simulink model "Trolley_Pendulum_RBF_Supervisory"  (R2023b)
settings: Solver=ode1  StartTime=0.0  StopTime=10  FixedStep=0.001  RelTol=1e-3
values from neighbouring files (symbols this model uses):
  E = C'*Q_bar*M    [inverted_pendulum.m]
  H = C'*Q_bar*C+R_bar    [inverted_pendulum.m]
  m_A_continue = double(subs(A_syms, [M, m, g, J, L, b], [M_, m_, g_, J_, L_, b_]))    [inverted_pendulum.m]
  m_B_continue = double(subs(B_syms, [M, m, g, J, L, b], [M_, m_, g_, J_, L_, b_]))    [inverted_pendulum.m]
  m_C_continue = C_syms    [inverted_pendulum.m]
  N = 20    [inverted_pendulum.m]
  Time_Step = 0.03    [inverted_pendulum.m]
  X = [x, x_dt, fai, fai_dt]    [inverted_pendulum.m]
  Y = [x, x_dt, fai, fai_dt]    [inverted_pendulum.m]
undefined symbols (not defined in the file or in its folder): K, Z
libraries: sm_lib x16, nesl_utility x6, rllib x1
settings Model: Creator=Lenovo  LastModifiedBy=15324
settings SolverCC: AlgebraicLoopSolver=TrustRegion
settings DataIOCC: LimitDataPoints=on  SaveFormat=Array  ReturnWorkspaceOutputs=off
settings OptimizationCC: BlockReduction=off  BooleanDataType=off  LifeSpan=inf
settings DebuggingCC: SaveWithParameterizedLinksMsg=none  UnderspecifiedInitializationDetection=Classic  MergeDetectMultiDrivingBlocksExec=none  SignalResolutionControl=TryResolveAllWithWarning  UnconnectedInputMsg=warning  UnconnectedOutputMsg=warning  UnconnectedLineMsg=warning  SFUnexpectedBacktrackingDiag=warning  SFNoUnconditionalDefaultTransitionDiag=warning  SFExecutionAtInitializationDiag=none  ArithmeticOperatorsInVariantConditions=warning
settings HardwareCC: ProdBitPerPointer=32  ProdBitPerSizeT=32  ProdBitPerPtrDiffT=32  ProdLargestAtomicFloat=None  ProdIntDivRoundTo=Undefined  ProdEndianess=Unspecified  ProdWordSize=32  ProdHWDeviceType=32-bit Generic  TargetUnknown=on
settings ModelReferenceCC: EnableRefExpFcnMdlSchedulingChecks=on  PropagateSignalLabelsOutOfModel=off
settings SFSimCC: SimUseLocalCustomCode=off  CustomCodeUndefinedFunction=UseInterfaceOnly
settings RTWCC: RTWUseLocalCustomCode=off
settings CodeAppCC: StateflowObjectComments=on
settings GRTTargetCC: TargetLangStandard=C89/C90 (ANSI)
settings ConfigComp: CovMetricSettings=dw  CovSaveCumulativeToWorkspaceVar=on  CovSaveSingleToWorkspaceVar=on  CovExternalEMLEnable=off

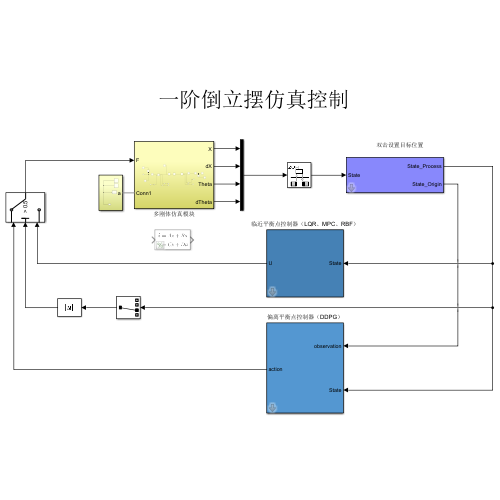
[thumbnail: Simulink's stored preview of the top-level diagram]
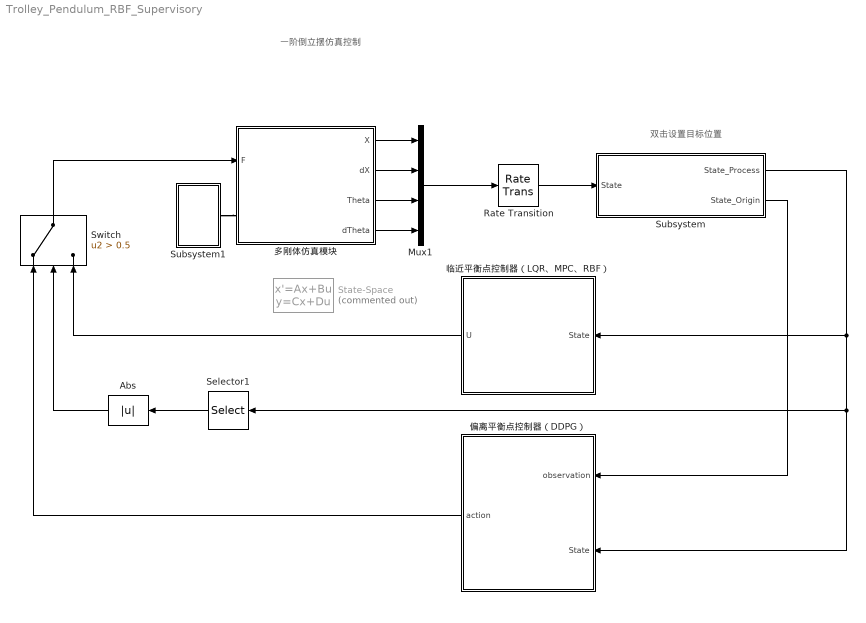
== system Trolley_Pendulum_RBF_Supervisory ==
  note: 双击设置目标位置
  note: 一阶倒立摆仿真控制
  Abs : Abs  SaturateOnIntegerOverflow=off
  Mux1 : Mux
  Rate Transition : RateTransition  OutPortSampleTime=Time_Step
  Selector1 : Selector  InputPortWidth=4  IndexOptions=Index vector (dialog)  Indices=[3]  OutputSizes=1
  State-Space : StateSpace  Commented=on  A=m_A_continue  B=m_B_continue  C=m_C_continue  D=[0;0;0;0]  InitialCondition=[0.5;0.5;0.5;0.5]
  Subsystem : Subsystem  mask{X_Target=1}
      mask prompts: X_Target "目标位置"
      mask DialogControl Set Prompt: 设置
  Subsystem1 : Subsystem
  Switch : Switch  Criteria=u2 > Threshold  Threshold=0.5  SaturateOnIntegerOverflow=off  InputSameDT=off
  临近平衡点控制器（LQR、MPC、RBF） : Subsystem  mask{MODE=MPC}
      mask prompts: MODE "模式设置"
      mask TypeOptions MODE: MPC | LQR | RBF
      mask DialogControl ParameterGroupVar Prompt: 设置
      mask DialogControl MODE Tooltip: A
  偏离平衡点控制器（DDPG） : Subsystem
      mask DialogControl ParameterGroupVar Prompt: 基于强化学习DDPG控制器
  多刚体仿真模块 : Subsystem
  wires:
  多刚体仿真模块/2(dX) -> Mux1/2
  Mux1/1 -> Rate Transition/1
  多刚体仿真模块/4(dTheta) -> Mux1/4
  多刚体仿真模块/1(X) -> Mux1/1
  多刚体仿真模块/3(Theta) -> Mux1/3
  Abs/1 -> Switch/2
  Selector1/1 -> Abs/1
  Switch/1 -> 多刚体仿真模块/1(F)
  Subsystem/1(State_Process) -> 偏离平衡点控制器（DDPG）/2(State), Selector1/1, 临近平衡点控制器（LQR、MPC、RBF）/1(State)
  Rate Transition/1 -> Subsystem/1(State)
  偏离平衡点控制器（DDPG）/1(action) -> Switch/1
  Subsystem/2(State_Origin) -> 偏离平衡点控制器（DDPG）/1(observation)
  临近平衡点控制器（LQR、MPC、RBF）/1(U) -> Switch/3
  connections:
  Subsystem1/RConn1 -- 多刚体仿真模块/LConn1

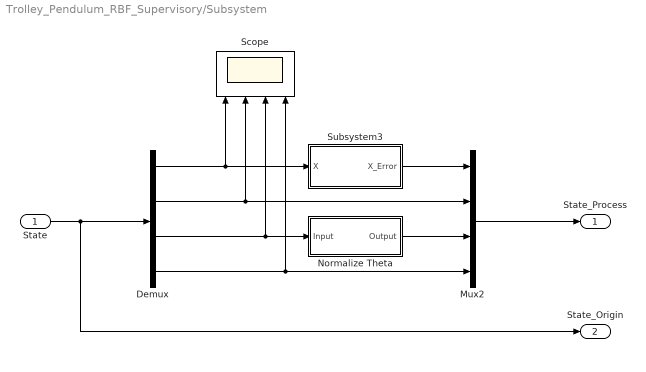
== system Trolley_Pendulum_RBF_Supervisory/Subsystem ==
  State : Inport
  Demux : Demux
  Mux2 : Mux
  Normalize Theta : Subsystem
  Scope : Scope  NumInputPorts=4
  Subsystem3 : Subsystem  mask{POS_REF=X_Target}
      mask prompts: POS_REF "目标位置"
      mask DialogControl ParameterGroupVar Prompt: 参数
  State_Process : Outport
  State_Origin : Outport  Port=2
  wires:
  Mux2/1 -> State_Process/1
  State/1 -> State_Origin/1, Demux/1
  Demux/2 -> Scope/2, Mux2/2
  Normalize Theta/1(Output) -> Mux2/3
  Demux/3 -> Scope/3, Normalize Theta/1(Input)
  Demux/4 -> Scope/4, Mux2/4
  Demux/1 -> Scope/1, Subsystem3/1(X)
  Subsystem3/1(X_Error) -> Mux2/1

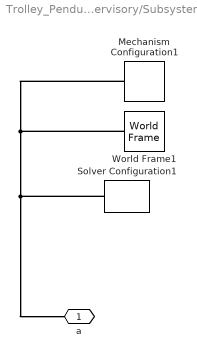
== system Trolley_Pendulum_RBF_Supervisory/Subsystem1 ==
  Mechanism Configuration1 : sm_lib/Utilities/Mechanism Configuration  UniformGravity=Constant  GravityVector=[0 0 -9.80665]  GravityVectorUnits=m/s^2  LinearizationDelta=0.0001  JointModeTransitionNonlinearIterations=2
  Solver Configuration1 : nesl_utility/Solver Configuration  PhysicalDomain=network_engine_domain  SubClassName=solver  LeftPortType=input  RightPortType=generic  Tones=[]  Harmonics=[]  SimulateNoise=off  Profile=off  UseLocalSampling=off  EnableSwitchedLinearOptims=on  FrequencyDomain=off  UseCCode=off  RelTol=0.001  AbsTol=1e-06  MinStep=1e-09  ToWorkspace=off  RevertToSquareIcSolve=off  NumHomotopyIterations=100  PhasorMode=off  PhasorModeNumHarmonics=1  ConsistencySolver=NEWTON_FTOL  IndexReductionMethod=DerivativeReplacement  DoDC=off  ResidualTolerance=1e-09  ConsistencyTolSource=GLOBAL  ConsistencyAbsTol=0.001  ConsistencyRelTol=0.001  ConsistencyTolFactor=0.001  UseLocalSolver=off  LocalSolverChoice=NE_BACKWARD_EULER_ADVANCER  ResolveIndetEquations=on  FunctionEvalNumThread=1  LocalSolverSampleTime=0.001  DoFixedCost=off  MaxNonlinIter=3  MaxModeIter=2  ComputeImpulses=off  ImpulseIterations=2  LinearAlgebra=auto  LinearAlgebraNumThread=0  EquationFormulation=NE_TIME_EF  DelaysMemoryBudget=1024  AutomaticFiltering=on  FilteringTimeConstant=0.001  PartitionStorageMethod=AS_NEEDED  PartitionMemoryBudget=1024  PartitionMethod=ROBUST  MultibodyUseLocalSolver=off  MultibodyLocalSolverChoice=ODE1  MultibodyLocalSolverSampleTime=0.001
  World Frame1 : sm_lib/Frames and Transforms/World Frame
  a : PMIOPort  Side=Right
  connections:
  Mechanism Configuration1/RConn1 -- a/RConn1 -- Solver Configuration1/RConn1 -- World Frame1/RConn1

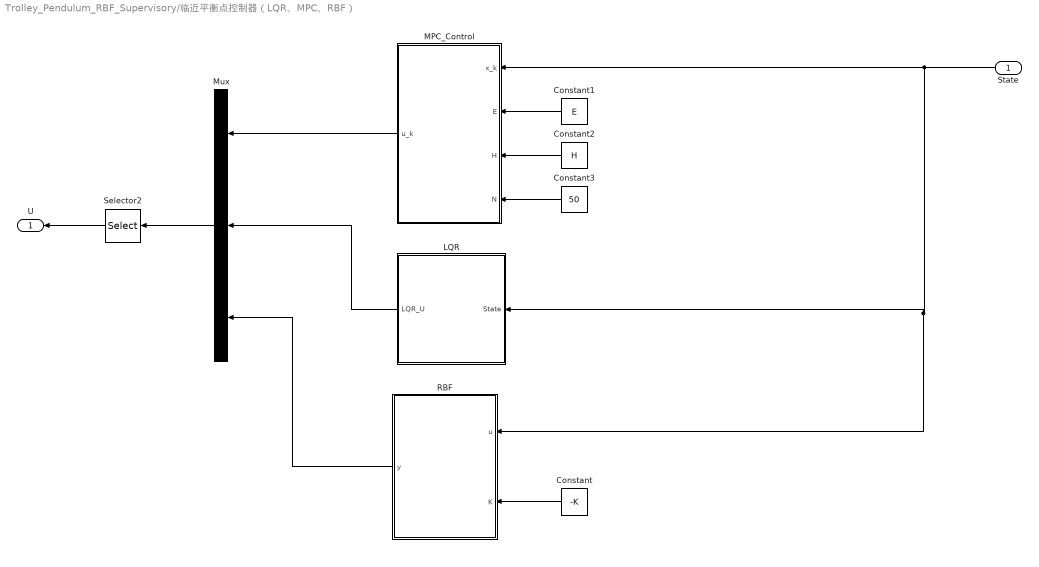
== system Trolley_Pendulum_RBF_Supervisory/临近平衡点控制器（LQR、MPC、RBF） ==
  State : Inport
  Constant : Constant  Value=-K  VectorParams1D=off
  Constant1 : Constant  Value=E  VectorParams1D=off
  Constant2 : Constant  Value=H  VectorParams1D=off
  Constant3 : Constant  Value=50
  LQR : Subsystem  mask{LQR_K=K}
      mask prompts: LQR_K "LQR_K矩阵"
      mask DialogControl ParameterGroupVar Prompt: 参数
  MPC_Control : MATLAB Function  TreatAsAtomicUnit=on
  Mux : Mux  Inputs=3
  RBF : MATLAB Function  TreatAsAtomicUnit=on
  Selector2 : Selector  InputPortWidth=3  IndexOptions=Index vector (dialog)  Indices=[MODE]  OutputSizes=1
  U : Outport
  wires:
  Selector2/1 -> U/1
  LQR/1(LQR_U) -> Mux/2
  MPC_Control/1(u_k) -> Mux/1
  Mux/1 -> Selector2/1
  Constant1/1 -> MPC_Control/2(E)
  Constant/1 -> RBF/2(K)
  RBF/1(y) -> Mux/3
  Constant2/1 -> MPC_Control/3(H)
  Constant3/1 -> MPC_Control/4(N)
  State/1 -> RBF/1(u), LQR/1(State), MPC_Control/1(x_k)

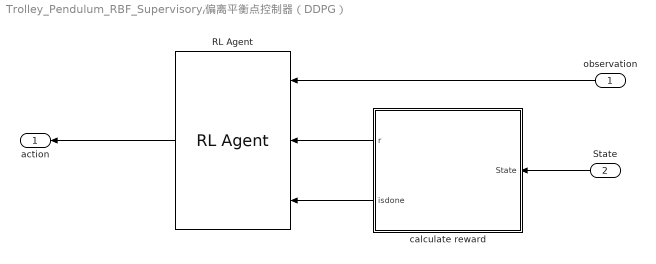
== system Trolley_Pendulum_RBF_Supervisory/偏离平衡点控制器（DDPG） ==
  observation : Inport
  State : Inport  Port=2
  RL Agent : rllib/RL Agent  Agent=saved_agent  ExternalActionAsInput=off  ProvideLastAction=off  ProvideCumRwd=off  TreatAsDirectFeedthrough=on  UseStrictObservationDataTypes=off
  calculate reward : Subsystem
  action : Outport
  wires:
  observation/1 -> RL Agent/1
  calculate reward/2(isdone) -> RL Agent/3
  calculate reward/1(r) -> RL Agent/2
  State/1 -> calculate reward/1(State)
  RL Agent/1 -> action/1

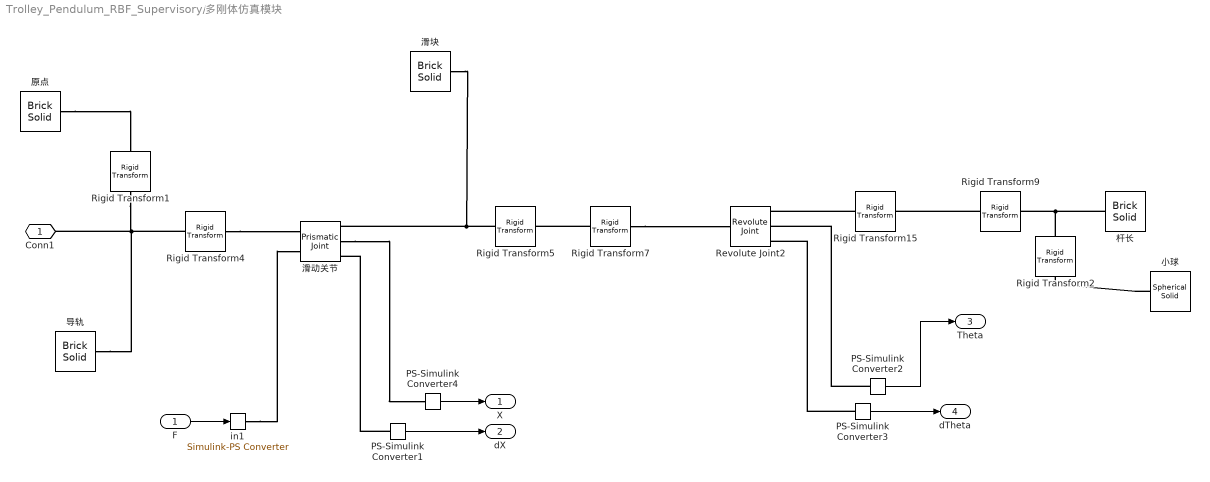
== system Trolley_Pendulum_RBF_Supervisory/多刚体仿真模块 ==
  F : Inport
  PS-Simulink Converter1 : nesl_utility/PS-Simulink Converter  PhysicalDomain=network_engine_domain  SubClassName=ps_output  LeftPortType=input  RightPortType=output  PseudoPeriodic=off  Frequencies=[]  VectorFormat=inherit  Unit=m/s  AffineConversion=off
  PS-Simulink Converter2 : nesl_utility/PS-Simulink Converter  PhysicalDomain=network_engine_domain  SubClassName=ps_output  LeftPortType=input  RightPortType=output  PseudoPeriodic=off  Frequencies=[]  VectorFormat=inherit  Unit=rad  AffineConversion=off
  PS-Simulink Converter3 : nesl_utility/PS-Simulink Converter  PhysicalDomain=network_engine_domain  SubClassName=ps_output  LeftPortType=input  RightPortType=output  PseudoPeriodic=off  Frequencies=[]  VectorFormat=inherit  Unit=rad/s  AffineConversion=off
  PS-Simulink Converter4 : nesl_utility/PS-Simulink Converter  PhysicalDomain=network_engine_domain  SubClassName=ps_output  LeftPortType=input  RightPortType=output  PseudoPeriodic=off  Frequencies=[]  VectorFormat=inherit  Unit=m  AffineConversion=off
  Revolute Joint2 : sm_lib/Joints/Revolute Joint  JointMode=Normal  SenseConstraintForce=off  SenseConstraintForceX=off  SenseConstraintForceY=off  SenseConstraintForceZ=off  SenseConstraintTorque=off  SenseConstraintTorqueX=off  SenseConstraintTorqueY=off  SenseConstraintTorqueZ=off  SenseTotalForce=off  SenseTotalForceX=off  SenseTotalForceY=off  SenseTotalForceZ=off  SenseTotalTorque=off  SenseTotalTorqueX=off  SenseTotalTorqueY=off  SenseTotalTorqueZ=off  CompositeWrenchDir=FollowerOnBase  CompositeWrenchFrame=BaseFrame  EquilibriumPosition=0  EquilibriumPositionUnits=deg  SpringStiffness=0  SpringStiffnessUnits=N*m/deg  DampingCoefficient=0  DampingCoefficientUnits=N*m/(deg/s)  TorqueActuationMode=NoTorque  MotionActuationMode=ComputedMotion  SensePosition=on  SenseVelocity=on  SenseAcceleration=off  SenseTorqueForce=off  SenseLowerLimitTorqueForce=off  SenseUpperLimitTorqueForce=off  LowerLimitSpecify=off  LowerLimitBound=-90  LowerLimitBoundUnits=deg  LowerLimitStiffness=1e4  LowerLimitStiffnessUnits=N*m/deg  LowerLimitDamping=10  LowerLimitDampingUnits=N*m/(deg/s)  LowerLimitTransitionRegionWidth=0.1  LowerLimitTransitionRegionWidthUnits=deg  UpperLimitSpecify=off  UpperLimitBound=90  UpperLimitBoundUnits=deg  UpperLimitStiffness=1e4  UpperLimitStiffnessUnits=N*m/deg  UpperLimitDamping=10  UpperLimitDampingUnits=N*m/(deg/s)  UpperLimitTransitionRegionWidth=0.1  UpperLimitTransitionRegionWidthUnits=deg  PositionTargetSpecify=on  PositionTargetPriority=High  PositionTargetValue=150  PositionTargetValueUnits=deg  VelocityTargetSpecify=off  VelocityTargetPriority=High  VelocityTargetValue=0  VelocityTargetValueUnits=deg/s
  Rigid Transform1 : sm_lib/Frames and Transforms/Rigid Transform  TranslationMethod=None  TranslationStandardOffset=0  TranslationStandardOffsetUnits=m  TranslationStandardAxis=+Z  TranslationCartesianOffset=[0 0 0]  TranslationCartesianOffsetUnits=m  TranslationROffset=0  TranslationROffsetUnits=m  TranslationZOffset=0  TranslationZOffsetUnits=m  TranslationThetaOffset=0  TranslationThetaOffsetUnits=deg  RotationMethod=StandardAxis  RotationAngleUnits=deg  RotationStandardAxis=+Y  RotationAngle=90  RotationArbitraryAxis=[0 0 1]  FollAlignAxisA=+X  BaseAlignAxisA=+Y  FollAlignAxisB=+Y  BaseAlignAxisB=+Z  RotationSequenceAxes=FollowerAxes  RotationSequence=XYX  RotationSequenceAngles=[0 0 0]  RotationSequenceAnglesUnits=deg  RotationMatrix=[1 0 0; 0 1 0; 0 0 1]  Quaternion=[1 0 0 0]
  Rigid Transform15 : sm_lib/Frames and Transforms/Rigid Transform  TranslationMethod=None  TranslationStandardOffset=0  TranslationStandardOffsetUnits=m  TranslationStandardAxis=+Z  TranslationCartesianOffset=[0 0 0]  TranslationCartesianOffsetUnits=m  TranslationROffset=0  TranslationROffsetUnits=m  TranslationZOffset=0  TranslationZOffsetUnits=m  TranslationThetaOffset=0  TranslationThetaOffsetUnits=deg  RotationMethod=StandardAxis  RotationAngleUnits=deg  RotationStandardAxis=+X  RotationAngle=-90  RotationArbitraryAxis=[0 0 1]  FollAlignAxisA=+X  BaseAlignAxisA=+Y  FollAlignAxisB=+Y  BaseAlignAxisB=+Z  RotationSequenceAxes=FollowerAxes  RotationSequence=XYX  RotationSequenceAngles=[0 0 0]  RotationSequenceAnglesUnits=deg  RotationMatrix=[1 0 0; 0 1 0; 0 0 1]  Quaternion=[1 0 0 0]
  Rigid Transform2 : sm_lib/Frames and Transforms/Rigid Transform  TranslationMethod=StandardAxis  TranslationStandardOffset=25  TranslationStandardOffsetUnits=cm  TranslationStandardAxis=+Z  TranslationCartesianOffset=[0 0 0]  TranslationCartesianOffsetUnits=cm  TranslationROffset=0  TranslationROffsetUnits=m  TranslationZOffset=0  TranslationZOffsetUnits=m  TranslationThetaOffset=0  TranslationThetaOffsetUnits=deg  RotationMethod=None  RotationAngleUnits=deg  RotationStandardAxis=+X  RotationAngle=90  RotationArbitraryAxis=[0 0 1]  FollAlignAxisA=+X  BaseAlignAxisA=+Y  FollAlignAxisB=+Y  BaseAlignAxisB=+Z  RotationSequenceAxes=FollowerAxes  RotationSequence=XYX  RotationSequenceAngles=[0 0 0]  RotationSequenceAnglesUnits=deg  RotationMatrix=[1 0 0; 0 1 0; 0 0 1]  Quaternion=[1 0 0 0]
  Rigid Transform4 : sm_lib/Frames and Transforms/Rigid Transform  TranslationMethod=None  TranslationStandardOffset=0  TranslationStandardOffsetUnits=m  TranslationStandardAxis=+Z  TranslationCartesianOffset=[0 0 0]  TranslationCartesianOffsetUnits=m  TranslationROffset=0  TranslationROffsetUnits=m  TranslationZOffset=0  TranslationZOffsetUnits=m  TranslationThetaOffset=0  TranslationThetaOffsetUnits=deg  RotationMethod=StandardAxis  RotationAngleUnits=deg  RotationStandardAxis=+Y  RotationAngle=90  RotationArbitraryAxis=[0 0 1]  FollAlignAxisA=+X  BaseAlignAxisA=+Y  FollAlignAxisB=+Y  BaseAlignAxisB=+Z  RotationSequenceAxes=FollowerAxes  RotationSequence=XYX  RotationSequenceAngles=[0 0 0]  RotationSequenceAnglesUnits=deg  RotationMatrix=[1 0 0; 0 1 0; 0 0 1]  Quaternion=[1 0 0 0]
  Rigid Transform5 : sm_lib/Frames and Transforms/Rigid Transform  TranslationMethod=None  TranslationStandardOffset=0  TranslationStandardOffsetUnits=m  TranslationStandardAxis=+Z  TranslationCartesianOffset=[0 0 0]  TranslationCartesianOffsetUnits=m  TranslationROffset=0  TranslationROffsetUnits=m  TranslationZOffset=0  TranslationZOffsetUnits=m  TranslationThetaOffset=0  TranslationThetaOffsetUnits=deg  RotationMethod=StandardAxis  RotationAngleUnits=deg  RotationStandardAxis=+Y  RotationAngle=-90  RotationArbitraryAxis=[0 0 1]  FollAlignAxisA=+X  BaseAlignAxisA=+Y  FollAlignAxisB=+Y  BaseAlignAxisB=+Z  RotationSequenceAxes=FollowerAxes  RotationSequence=XYX  RotationSequenceAngles=[0 0 0]  RotationSequenceAnglesUnits=deg  RotationMatrix=[1 0 0; 0 1 0; 0 0 1]  Quaternion=[1 0 0 0]
  Rigid Transform7 : sm_lib/Frames and Transforms/Rigid Transform  TranslationMethod=None  TranslationStandardOffset=0  TranslationStandardOffsetUnits=m  TranslationStandardAxis=+Z  TranslationCartesianOffset=[0 0 0]  TranslationCartesianOffsetUnits=m  TranslationROffset=0  TranslationROffsetUnits=m  TranslationZOffset=0  TranslationZOffsetUnits=m  TranslationThetaOffset=0  TranslationThetaOffsetUnits=deg  RotationMethod=StandardAxis  RotationAngleUnits=deg  RotationStandardAxis=+X  RotationAngle=+90  RotationArbitraryAxis=[0 0 1]  FollAlignAxisA=+X  BaseAlignAxisA=+Y  FollAlignAxisB=+Y  BaseAlignAxisB=+Z  RotationSequenceAxes=FollowerAxes  RotationSequence=XYX  RotationSequenceAngles=[0 0 0]  RotationSequenceAnglesUnits=deg  RotationMatrix=[1 0 0; 0 1 0; 0 0 1]  Quaternion=[1 0 0 0]
  Rigid Transform9 : sm_lib/Frames and Transforms/Rigid Transform  TranslationMethod=StandardAxis  TranslationStandardOffset=25  TranslationStandardOffsetUnits=cm  TranslationStandardAxis=+Z  TranslationCartesianOffset=[0 0 0]  TranslationCartesianOffsetUnits=cm  TranslationROffset=0  TranslationROffsetUnits=m  TranslationZOffset=0  TranslationZOffsetUnits=m  TranslationThetaOffset=0  TranslationThetaOffsetUnits=deg  RotationMethod=None  RotationAngleUnits=deg  RotationStandardAxis=+X  RotationAngle=90  RotationArbitraryAxis=[0 0 1]  FollAlignAxisA=+X  BaseAlignAxisA=+Y  FollAlignAxisB=+Y  BaseAlignAxisB=+Z  RotationSequenceAxes=FollowerAxes  RotationSequence=XYX  RotationSequenceAngles=[0 0 0]  RotationSequenceAnglesUnits=deg  RotationMatrix=[1 0 0; 0 1 0; 0 0 1]  Quaternion=[1 0 0 0]
  in1 : nesl_utility/Simulink-PS Converter  PhysicalDomain=network_engine_domain  SubClassName=ps_input  LeftPortType=input  RightPortType=output  PseudoPeriodic=off  Frequencies=[]  NoiseDistribution=none  NoiseParameters=[]  Unit=1  AffineConversion=off  FilteringAndDerivatives=provide  SimscapeFilterOrder=1  InputFilterTimeConstant=0.001  UdotUserProvided=0
  原点 : sm_lib/Body Elements/Brick Solid  GraphicAmbientColor=[0.15 0.15 0.15 1.0]  BasedOnType=Density  BrickDimensions=[5 11 5]  BrickDimensionsUnits=cm  CenterOfMass=[0 0 0]  CenterOfMassUnits=m  GraphicDiffuseColor=[0.3 0.8 0.5]  Density=0.1  DensityUnits=g/cm^3  DoExposeReferenceFrame=on  GraphicEmissiveColor=[0.0 0.0 0.0 1.0]  ExportEntireGeometry=off  SerializedFrames=<Frames/>  MarkerShape=Sphere  MarkerSize=10  GraphicType=FromGeometry  InertiaType=CalculateFromGeometry  Mass=1  MassUnits=kg  MomentsOfInertia=[1 1 1]  MomentsOfInertiaUnits=kg*m^2  GraphicOpacity=1.0  ProductsOfInertia=[0 0 0]  ProductsOfInertiaUnits=kg*m^2  GraphicShininess=75  GraphicSpecularColor=[0.5 0.5 0.5 1.0]  GraphicVisPropType=SimpleVisualProperties
  导轨 : sm_lib/Body Elements/Brick Solid  GraphicAmbientColor=[0.15 0.15 0.15 1.0]  BasedOnType=Density  BrickDimensions=[500 5 5]  BrickDimensionsUnits=cm  CenterOfMass=[0 0 0]  CenterOfMassUnits=m  GraphicDiffuseColor=[0 0 0]  Density=0.1  DensityUnits=g/cm^3  DoExposeReferenceFrame=on  GraphicEmissiveColor=[0.0 0.0 0.0 1.0]  ExportEntireGeometry=off  SerializedFrames=<Frames/>  MarkerShape=Sphere  MarkerSize=10  GraphicType=FromGeometry  InertiaType=CalculateFromGeometry  Mass=1  MassUnits=kg  MomentsOfInertia=[1 1 1]  MomentsOfInertiaUnits=kg*m^2  GraphicOpacity=1.0  ProductsOfInertia=[0 0 0]  ProductsOfInertiaUnits=kg*m^2  GraphicShininess=75  GraphicSpecularColor=[0.5 0.5 0.5 1.0]  GraphicVisPropType=SimpleVisualProperties
  小球 : sm_lib/Body Elements/Spherical Solid  GraphicAmbientColor=[0.15 0.15 0.15 1.0]  BasedOnType=Density  CenterOfMass=[0 0 0]  CenterOfMassUnits=m  GraphicDiffuseColor=[0.5 0.8 0.5]  Density=1  DensityUnits=kg/m^3  DoExposeReferenceFrame=on  GraphicEmissiveColor=[0.0 0.0 0.0 1.0]  ExportEntireGeometry=off  SerializedExposedGeometries=<exposedGeometries/>  SerializedFrames=<Frames/>  MarkerShape=Sphere  MarkerSize=10  GraphicType=FromGeometry  InertiaType=CalculateFromGeometry  Mass=1  MassUnits=kg  MomentsOfInertia=[1 1 1]  MomentsOfInertiaUnits=kg*m^2  GraphicOpacity=1.0  ProductsOfInertia=[0 0 0]  ProductsOfInertiaUnits=kg*m^2  GraphicShininess=75  GraphicSpecularColor=[0.5 0.5 0.5 1.0]  SphereRadius=3.5  SphereRadiusUnits=cm  GraphicVisPropType=SimpleVisualProperties
  杆长 : sm_lib/Body Elements/Brick Solid  GraphicAmbientColor=[0.15 0.15 0.15 1.0]  BasedOnType=Density  BrickDimensions="[5 5  50]"  BrickDimensionsUnits=cm  CenterOfMass=[0 0 0]  CenterOfMassUnits=m  GraphicDiffuseColor=[0.8 0.5 0.1]  Density=1  DensityUnits=g/cm^3  DoExposeReferenceFrame=on  GraphicEmissiveColor=[0.0 0.0 0.0 1.0]  ExportEntireGeometry=off  SerializedFrames=<Frames/>  MarkerShape=Sphere  MarkerSize=10  GraphicType=FromGeometry  InertiaType=CalculateFromGeometry  Mass=1  MassUnits=kg  MomentsOfInertia=[1 1 1]  MomentsOfInertiaUnits=kg*m^2  GraphicOpacity=1.0  ProductsOfInertia=[0 0 0]  ProductsOfInertiaUnits=kg*m^2  GraphicShininess=75  GraphicSpecularColor=[0.5 0.5 0.5 1.0]  GraphicVisPropType=SimpleVisualProperties
  滑动关节 : sm_lib/Joints/Prismatic Joint  JointMode=Normal  SenseConstraintForce=off  SenseConstraintForceX=off  SenseConstraintForceY=off  SenseConstraintForceZ=off  SenseConstraintTorque=off  SenseConstraintTorqueX=off  SenseConstraintTorqueY=off  SenseConstraintTorqueZ=off  SenseTotalForce=off  SenseTotalForceX=off  SenseTotalForceY=off  SenseTotalForceZ=off  SenseTotalTorque=off  SenseTotalTorqueX=off  SenseTotalTorqueY=off  SenseTotalTorqueZ=off  CompositeWrenchDir=FollowerOnBase  CompositeWrenchFrame=BaseFrame  EquilibriumPosition=0  EquilibriumPositionUnits=m  SpringStiffness=0  SpringStiffnessUnits=N/m  DampingCoefficient=0  DampingCoefficientUnits=N/(m/s)  TorqueActuationMode=InputTorque  MotionActuationMode=ComputedMotion  SensePosition=on  SenseVelocity=on  SenseAcceleration=off  SenseTorqueForce=off  SenseLowerLimitTorqueForce=off  SenseUpperLimitTorqueForce=off  LowerLimitSpecify=off  LowerLimitBound=-1  LowerLimitBoundUnits=m  LowerLimitStiffness=1e6  LowerLimitStiffnessUnits=N/m  LowerLimitDamping=1e3  LowerLimitDampingUnits=N/(m/s)  LowerLimitTransitionRegionWidth=1e-4  LowerLimitTransitionRegionWidthUnits=m  UpperLimitSpecify=off  UpperLimitBound=1  UpperLimitBoundUnits=m  UpperLimitStiffness=1e6  UpperLimitStiffnessUnits=N/m  UpperLimitDamping=1e3  UpperLimitDampingUnits=N/(m/s)  UpperLimitTransitionRegionWidth=1e-4  UpperLimitTransitionRegionWidthUnits=m  PositionTargetSpecify=off  PositionTargetPriority=High  PositionTargetValue=0  PositionTargetValueUnits=m  VelocityTargetSpecify=off  VelocityTargetPriority=High  VelocityTargetValue=0  VelocityTargetValueUnits=m/s
  滑块 : sm_lib/Body Elements/Brick Solid  GraphicAmbientColor=[0.15 0.15 0.15 1.0]  BasedOnType=Density  BrickDimensions=[10 10 10]  BrickDimensionsUnits=cm  CenterOfMass=[0 0 0]  CenterOfMassUnits=m  GraphicDiffuseColor=[0.1 0.1 0.8]  Density=1  DensityUnits=g/cm^3  DoExposeReferenceFrame=on  GraphicEmissiveColor=[0.0 0.0 0.0 1.0]  ExportEntireGeometry=off  SerializedFrames=<Frames/>  MarkerShape=Sphere  MarkerSize=10  GraphicType=FromGeometry  InertiaType=CalculateFromGeometry  Mass=1  MassUnits=kg  MomentsOfInertia=[1 1 1]  MomentsOfInertiaUnits=kg*m^2  GraphicOpacity=1.0  ProductsOfInertia=[0 0 0]  ProductsOfInertiaUnits=kg*m^2  GraphicShininess=75  GraphicSpecularColor=[0.5 0.5 0.5 1.0]  GraphicVisPropType=SimpleVisualProperties
  Conn1 : PMIOPort  Side=Left
  X : Outport
  dX : Outport  Port=2
  Theta : Outport  Port=3
  dTheta : Outport  Port=4
  wires:
  F/1 -> in1/1
  PS-Simulink Converter1/1 -> dX/1
  PS-Simulink Converter3/1 -> dTheta/1
  PS-Simulink Converter2/1 -> Theta/1
  PS-Simulink Converter4/1 -> X/1
  connections:
  Rigid Transform9/LConn1 -- Rigid Transform15/RConn1
  in1/RConn1 -- 滑动关节/LConn2
  Rigid Transform15/LConn1 -- Revolute Joint2/RConn1
  Rigid Transform7/RConn1 -- Revolute Joint2/LConn1
  杆长/RConn1 -- Rigid Transform2/LConn1 -- Rigid Transform9/RConn1
  PS-Simulink Converter3/LConn1 -- Revolute Joint2/RConn3
  Rigid Transform7/LConn1 -- Rigid Transform5/RConn1
  Rigid Transform4/RConn1 -- 滑动关节/LConn1
  PS-Simulink Converter2/LConn1 -- Revolute Joint2/RConn2
  Rigid Transform4/LConn1 -- Rigid Transform1/RConn1 -- Conn1/RConn1 -- 导轨/RConn1
  PS-Simulink Converter1/LConn1 -- 滑动关节/RConn3
  滑动关节/RConn2 -- PS-Simulink Converter4/LConn1
  原点/RConn1 -- Rigid Transform1/LConn1
  小球/RConn1 -- Rigid Transform2/RConn1
  Rigid Transform5/LConn1 -- 滑块/RConn1 -- 滑动关节/RConn1

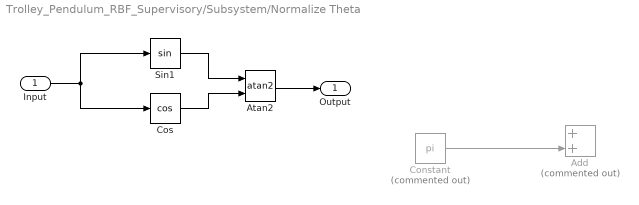
== system Trolley_Pendulum_RBF_Supervisory/Subsystem/Normalize Theta ==
  Input : Inport
  Add : Sum  Commented=on
  Atan2 : Trigonometry  Operator=atan2
  Constant : Constant  Commented=on  Value=pi
  Cos : Trigonometry  Operator=cos
  Sin1 : Trigonometry
  Output : Outport
  wires:
  Input/1 -> Cos/1, Sin1/1
  Sin1/1 -> Atan2/1
  Cos/1 -> Atan2/2
  Atan2/1 -> Output/1
  Constant/1 -> Add/2

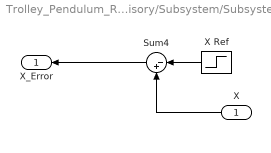
== system Trolley_Pendulum_RBF_Supervisory/Subsystem/Subsystem3 ==
  X : Inport
  Sum4 : Sum  Inputs=|-+
  X Ref : Step  Time=0  After=POS_REF  SampleTime=Time_Step
  X_Error : Outport
  wires:
  X Ref/1 -> Sum4/1
  X/1 -> Sum4/2
  Sum4/1 -> X_Error/1

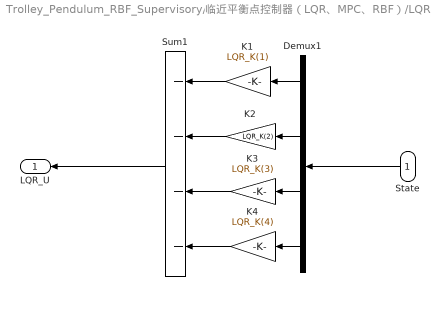
== system Trolley_Pendulum_RBF_Supervisory/临近平衡点控制器（LQR、MPC、RBF）/LQR ==
  State : Inport
  Demux1 : Demux
  K1 : Gain  Gain=LQR_K(1)
  K2 : Gain  Gain=LQR_K(2)
  K3 : Gain  Gain=LQR_K(3)
  K4 : Gain  Gain=LQR_K(4)
  Sum1 : Sum  Inputs=----
  LQR_U : Outport
  wires:
  K2/1 -> Sum1/2
  K1/1 -> Sum1/1
  K3/1 -> Sum1/3
  K4/1 -> Sum1/4
  Sum1/1 -> LQR_U/1
  State/1 -> Demux1/1
  Demux1/2 -> K2/1
  Demux1/3 -> K3/1
  Demux1/4 -> K4/1
  Demux1/1 -> K1/1

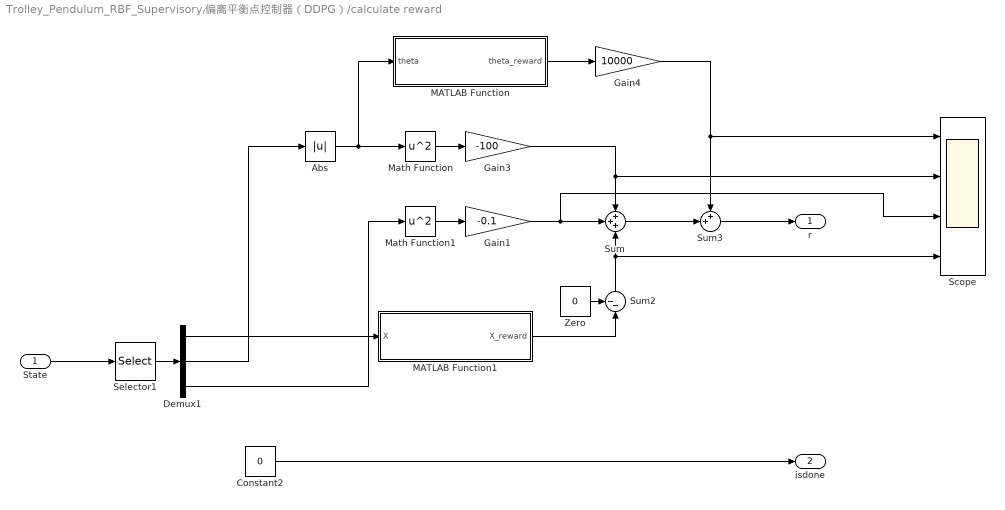
== system Trolley_Pendulum_RBF_Supervisory/偏离平衡点控制器（DDPG）/calculate reward ==
  State : Inport
  Abs : Abs  SaturateOnIntegerOverflow=off
  Constant2 : Constant  Value=0
  Demux1 : Demux  Outputs=3
  Gain1 : Gain  Gain=-0.1
  Gain3 : Gain  Gain=-100
  Gain4 : Gain  Gain=10000
  MATLAB Function : MATLAB Function  TreatAsAtomicUnit=on
  MATLAB Function1 : MATLAB Function  TreatAsAtomicUnit=on
  Math Function : Math  Operator=square  SignedPower=on
  Math Function1 : Math  Operator=square  SignedPower=on
  Scope : Scope  NumInputPorts=4
  Selector1 : Selector  InputPortWidth=4  IndexOptions=Index vector (dialog)  Indices=[1 3 4]  OutputSizes=1
  Sum : Sum  Inputs=+++
  Sum2 : Sum  Inputs=--|
  Sum3 : Sum  Inputs=++|
  Zero : Constant  Value=0  OutDataTypeStr=Inherit: Inherit via back propagation
  r : Outport
  isdone : Outport  Port=2
  wires:
  Math Function/1 -> Gain3/1
  Math Function1/1 -> Gain1/1
  Gain1/1 -> Scope/3, Sum/2
  Gain3/1 -> Scope/2, Sum/1
  Sum2/1 -> Scope/4, Sum/3
  Constant2/1 -> isdone/1
  Sum/1 -> Sum3/2
  Sum3/1 -> r/1
  Abs/1 -> MATLAB Function/1(theta), Math Function/1
  MATLAB Function/1(theta_reward) -> Gain4/1
  Gain4/1 -> Sum3/1, Scope/1
  Zero/1 -> Sum2/1
  MATLAB Function1/1(X_reward) -> Sum2/2
  State/1 -> Selector1/1
  Selector1/1 -> Demux1/1
  Demux1/1 -> MATLAB Function1/1(X)
  Demux1/2 -> Abs/1
  Demux1/3 -> Math Function1/1

== matlab function Trolley_Pendulum_RBF_Supervisory/临近平衡点控制器（LQR、MPC、RBF）/MPC_Control ==
  data: x_k input; u_k output; E input; H input; N input
function u_k = Prediction(x_k, E, H, N)  
    % 初始化输出  
    U_k = zeros(N*1, 1); % NP x 1  
    u_k = zeros(1, 1); % 指定 u_k 为固定大小 p x 1

    % 获取 H 矩阵的行列数
    [m, n] = size(H);

    % 根据 H 矩阵的列数定义初始向量 x0
    x0 = zeros(n, 1);
    % 使用quadprog函数求解优化问题  
    opts = optimoptions('quadprog','Algorithm','active-set');
    [U_k, ~, ~] = quadprog(H, E * x_k, [], [], [], [], [], [], x0, opts);
      
    % 取第一个结果  
    u_k = U_k(1, 1);  
end

== matlab function Trolley_Pendulum_RBF_Supervisory/临近平衡点控制器（LQR、MPC、RBF）/RBF ==
  settings: updateMethod=DISCRETE
  data: u input; y output; K input
function y = fcn(u, K)
    persistent w w_1 w_2 u_law			% 定义全局变量
    if isempty(w)							% 给全局变量赋初值
        w = ones(4,1);
        w_1=w;
        w_2=w_1;
        u_law = 0;
    end
    
    %定义初始输出数组
    y = ones(1,1);

    %神经网络参数赋初值 
    b = ones(4,1);
    ci = 0.5*[-5 -2 0 5];
    c = [ci;ci;ci;ci];
    xite = 0.010;
    alfa = 0.1;
    % K = [3.1623 5.6674 -44.3596 -8.2240];

    %获取当前 MATLAB Function 的输入，从simulink图可以看出来输入是u 
    x1 = u(1,1);
    x2 = u(2,1);
    x3 = u(3,1);
    x4 = u(4,1);
    x = [x1 x2 x3 x4]';
    
    % 计算当前RBF神经网络隐含层的输出
    h = zeros(4,1);
    for j = 1:1:4
        h(j) = exp(-norm(x-c(:,j))^2/(2*b(j)*b(j)));
    end

    % 计算当前LQR控制器的输出 
    u_LQR = K * x;

    % 计算神经网络控制器的输出和神经网络权值调整
    dw = zeros(4,1);
    dw = xite * u_LQR *h;
    w = w_1 + dw + alfa * (w_1 - w_2);
    w_2 = w_1;
    w_1 = w;

    % 计算当前RBF神经网络控制器的输出
    u_NN = w' * h;

    % 计算当前系统的最终控制量输出  
    u_law = u_NN + u_LQR;

    % % 输出控制律限幅度  
    % if u_law >= 10
    %  u_law = 10;
    % end
    % if u_law <= -10
    %  u_law = -10;
    % end 
    
    % % 算法输出
    % y(1) = u_law;
    % y(2) = u_NN;
    % y(3) = u_LQR;

    y = u_law;
    
end

== matlab function Trolley_Pendulum_RBF_Supervisory/偏离平衡点控制器（DDPG）/calculate reward/MATLAB Function ==
  data: theta input; theta_reward output
function theta_reward = fcn(theta)

if theta == 0
    theta_reward = 1;
else 
    theta_reward = 1 / theta;
end

== matlab function Trolley_Pendulum_RBF_Supervisory/偏离平衡点控制器（DDPG）/calculate reward/MATLAB Function1 ==
  data: X input; X_reward output
function X_reward = fcn(X)

if X > 3 || X <-3
    X_reward = X^2 * 2000;
else 
    X_reward = X^2 * 15;
end
